simulink model "xDes"  (R2017a)
settings: Solver=VariableStepAuto  StartTime=0.0  StopTime=50.0  RelTol=1e-3
settings Model: Creator=tlara  LastModifiedBy=tlara

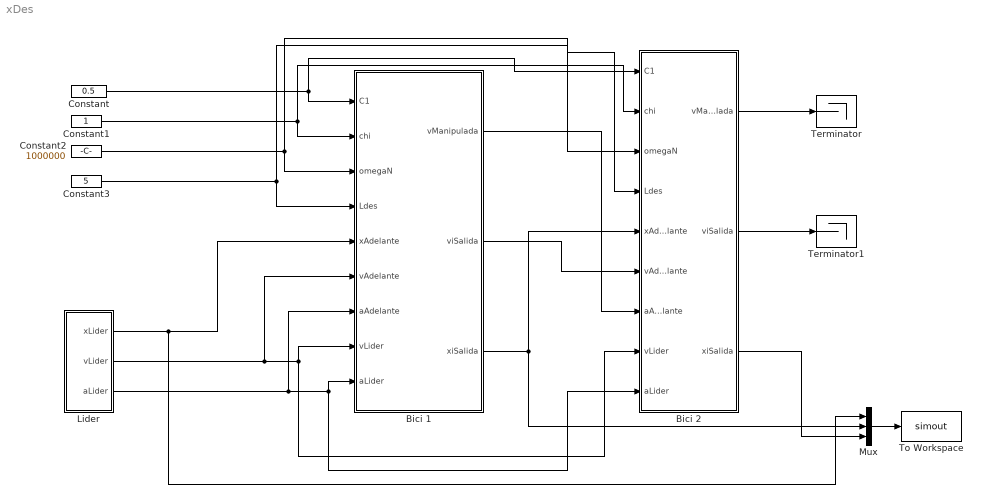
== system xDes ==
  Bici 1 : Subsystem
  Bici 2 : Subsystem
  Constant : Constant  Value=0.5
  Constant1 : Constant
  Constant2 : Constant  Value=1000000
  Constant3 : Constant  Value=5
  Lider : Subsystem
  Mux : Mux  Inputs=3
  Terminator : Terminator
  Terminator1 : Terminator
  To Workspace : ToWorkspace  VariableName=simout  SaveFormat=Timeseries  SampleTime=-1
  wires:
  Lider/1("xLider ") -> Mux/1, Bici 1/5(xAdelante)
  Bici 1/3("xiSalida ") -> Mux/2, Bici 2/5(xAdelante)
  Bici 1/2(viSalida) -> Bici 2/6(vAdelante)
  Bici 1/1(vManipulada) -> Bici 2/7(aAdelante)
  Lider/3("aLider ") -> Bici 1/7(aAdelante), Bici 2/9("aLider "), Bici 1/9("aLider ")
  Constant/1 -> Bici 2/1(C1), Bici 1/1(C1)
  Constant1/1 -> Bici 2/2(chi), Bici 1/2(chi)
  Constant2/1 -> Bici 2/3(omegaN), Bici 1/3(omegaN)
  Constant3/1 -> Bici 1/4(Ldes), Bici 2/4(Ldes)
  Bici 2/1(vManipulada) -> Terminator/1
  Bici 2/2(viSalida) -> Terminator1/1
  Lider/2(vLider) -> Bici 1/6(vAdelante), Bici 2/8("vLider "), Bici 1/8("vLider ")
  Bici 2/3("xiSalida ") -> Mux/3
  Mux/1 -> To Workspace/1

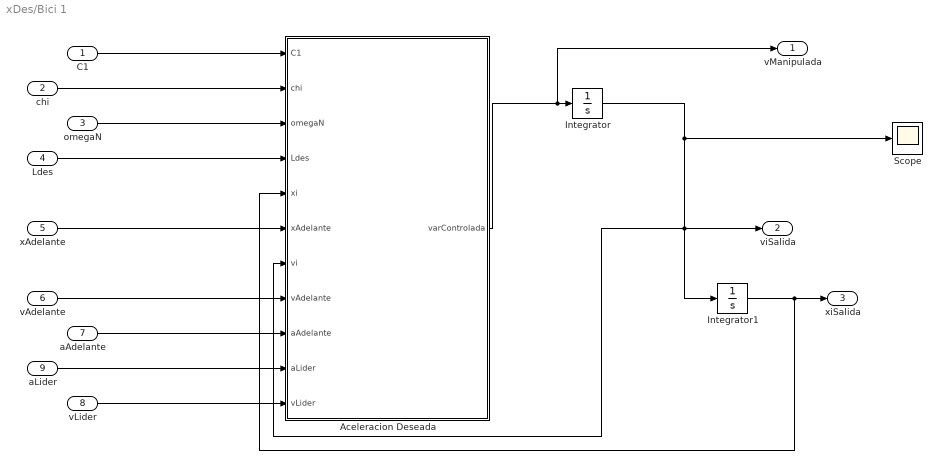
== system xDes/Bici 1 ==
  C1 : Inport
  chi : Inport  Port=2
  omegaN : Inport  Port=3
  Ldes : Inport  Port=4
  xAdelante : Inport  Port=5
  vAdelante : Inport  Port=6
  aAdelante : Inport  Port=7
  "vLider " : Inport  Port=8
  "aLider " : Inport  Port=9
  Aceleracion Deseada : MATLAB Function  TreatAsAtomicUnit=on
  Integrator : Integrator
  Integrator1 : Integrator  InitialCondition=10
  Scope : Scope
  vManipulada : Outport
  viSalida : Outport  Port=2
  "xiSalida " : Outport  Port=3
  wires:
  C1/1 -> Aceleracion Deseada/1(C1)
  "vLider "/1 -> Aceleracion Deseada/11(vLider)
  vAdelante/1 -> Aceleracion Deseada/8(vAdelante)
  "aLider "/1 -> Aceleracion Deseada/10(aLider)
  xAdelante/1 -> Aceleracion Deseada/6(xAdelante)
  aAdelante/1 -> Aceleracion Deseada/9(aAdelante)
  omegaN/1 -> Aceleracion Deseada/3(omegaN)
  Ldes/1 -> Aceleracion Deseada/4(Ldes)
  chi/1 -> Aceleracion Deseada/2(chi)
  Integrator1/1 -> Aceleracion Deseada/5(xi), "xiSalida "/1
  Aceleracion Deseada/1(varControlada) -> vManipulada/1, Integrator/1
  Integrator/1 -> Aceleracion Deseada/7(vi), Integrator1/1, viSalida/1, Scope/1

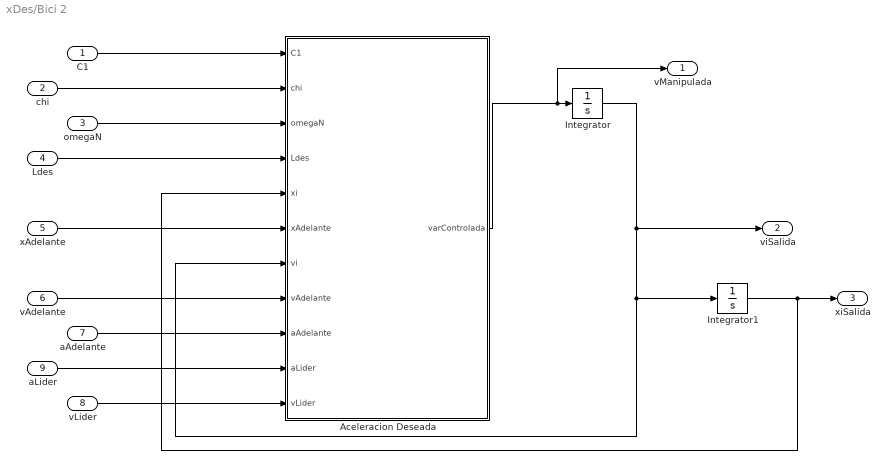
== system xDes/Bici 2 ==
  C1 : Inport
  chi : Inport  Port=2
  omegaN : Inport  Port=3
  Ldes : Inport  Port=4
  xAdelante : Inport  Port=5
  vAdelante : Inport  Port=6
  aAdelante : Inport  Port=7
  "vLider " : Inport  Port=8
  "aLider " : Inport  Port=9
  Aceleracion Deseada : MATLAB Function  TreatAsAtomicUnit=on
  Integrator : Integrator
  Integrator1 : Integrator
  vManipulada : Outport
  viSalida : Outport  Port=2
  "xiSalida " : Outport  Port=3
  wires:
  C1/1 -> Aceleracion Deseada/1(C1)
  "vLider "/1 -> Aceleracion Deseada/11(vLider)
  vAdelante/1 -> Aceleracion Deseada/8(vAdelante)
  "aLider "/1 -> Aceleracion Deseada/10(aLider)
  xAdelante/1 -> Aceleracion Deseada/6(xAdelante)
  aAdelante/1 -> Aceleracion Deseada/9(aAdelante)
  omegaN/1 -> Aceleracion Deseada/3(omegaN)
  Ldes/1 -> Aceleracion Deseada/4(Ldes)
  chi/1 -> Aceleracion Deseada/2(chi)
  Integrator1/1 -> Aceleracion Deseada/5(xi), "xiSalida "/1
  Aceleracion Deseada/1(varControlada) -> vManipulada/1, Integrator/1
  Integrator/1 -> Aceleracion Deseada/7(vi), Integrator1/1, viSalida/1

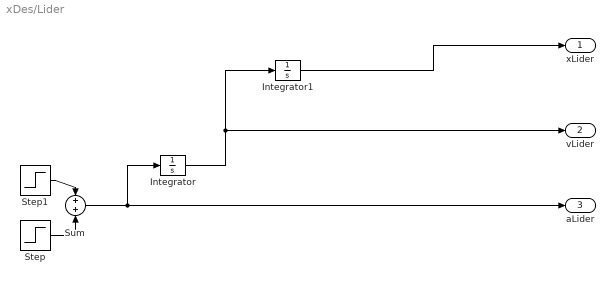
== system xDes/Lider ==
  Integrator : Integrator  InitialCondition=4.16
  Integrator1 : Integrator  InitialCondition=20
  Step : Step  Time=30  After=-0.1  SampleTime=0
  Step1 : Step  Time=20  After=0.1  SampleTime=0
  Sum : Sum
  "xLider " : Outport
  vLider : Outport  Port=2
  "aLider " : Outport  Port=3
  wires:
  Sum/1 -> Integrator/1, "aLider "/1
  Integrator/1 -> Integrator1/1, vLider/1
  Integrator1/1 -> "xLider "/1
  Step1/1 -> Sum/1
  Step/1 -> Sum/2

== matlab function xDes/Bici 1/Aceleracion Deseada ==
  data: C1 input; varControlada output; chi input; omegaN input; Ldes input; xi input; xAdelante input; vi input; vAdelante input; aAdelante input; aLider input; vLider input
function varControlada  = xDes(C1,chi,omegaN,Ldes,xi,xAdelante,vi,vAdelante,aAdelante,aLider,vLider)
%Constantes (Terminos que acompanan a los terminos de error.
alpha1 = 1-C1;
alpha2 = C1;
alpha3 = -1 * (2 * chi - C1* (chi + sqrt((chi^2) - 1))) * omegaN;
alpha4 = -1 * (chi + sqrt((chi^2) - 1)) * omegaN * C1;
alpha5 = -1 * (omegaN^2);

%Errores (epsilon)
errorSpacing =  xi - xAdelante + Ldes;
errorVelocidadRelativa = vi - vAdelante;

%Diferencia con el lider
difVLider = vi - vLider;

%Calculo del valor
varControlada = alpha1 * aAdelante + alpha2 * aLider + alpha3 * errorVelocidadRelativa + alpha4 * difVLider + alpha5 * errorSpacing;
vi = vi;
xi = xi;

== matlab function xDes/Bici 2/Aceleracion Deseada ==
  data: C1 input; varControlada output; chi input; omegaN input; Ldes input; xi input; xAdelante input; vi input; vAdelante input; aAdelante input; aLider input; vLider input
function varControlada  = xDes(C1,chi,omegaN,Ldes,xi,xAdelante,vi,vAdelante,aAdelante,aLider,vLider)
%Constantes (Terminos que acompanan a los terminos de error.
alpha1 = 1-C1;
alpha2 = C1;
alpha3 = -1 * (2 * chi - C1* (chi + sqrt((chi^2) - 1))) * omegaN;
alpha4 = -1 * (chi + sqrt((chi^2) - 1)) * omegaN * C1;
alpha5 = -1 * (omegaN^2);

%Errores (epsilon)
errorSpacing =  xi - xAdelante + Ldes;
errorVelocidadRelativa = vi - vAdelante;

%Diferencia con el lider
difVLider = vi - vLider;

%Calculo del valor
varControlada = alpha1 * aAdelante + alpha2 * aLider + alpha3 * errorVelocidadRelativa + alpha4 * difVLider + alpha5 * errorSpacing;
vi = vi;
xi = xi;
